simulink model "Amp_baseline"  (R2020a)
settings: Solver=ode45  StartTime=0.0  StopTime=inf  RelTol=1e-3
model workspace (MAT data in the model file):
  cfg_native : object (value not decoded)
  en_add_channels = 1
  host_ip = 2130706433
  host_port = 50223
  local_ip = 2130706433
  local_port = 50224
  num_en_channels = 32
  num_samples = 1
  sample_rate = 250
  serial_number = 'NB-2015.10.93'
undefined symbols (not defined in the file or in its folder): currentCFG_Amp_baseline_UB, UB
libraries: gtecHighspeedLib x7, gUSBamplib x1
settings Model: ModifiedByFormat=g.tec  Creator=g.tec medical engineering  LastModifiedBy=g.tec
settings DataIOCC: LimitDataPoints=on  SaveFormat=Array  ReturnWorkspaceOutputs=off
settings OptimizationCC: BlockReduction=off  BooleanDataType=off  LifeSpan=inf
settings DebuggingCC: SaveWithParameterizedLinksMsg=none  UnderspecifiedInitializationDetection=Classic  MergeDetectMultiDrivingBlocksExec=none  SignalResolutionControl=TryResolveAllWithWarning  FrameProcessingCompatibilityMsg=none  SFUnexpectedBacktrackingDiag=warning  SFNoUnconditionalDefaultTransitionDiag=warning  SFExecutionAtInitializationDiag=none  ArithmeticOperatorsInVariantConditions=warning
settings HardwareCC: ProdBitPerPointer=32  ProdBitPerSizeT=32  ProdBitPerPtrDiffT=32  ProdLargestAtomicFloat=None  ProdIntDivRoundTo=Undefined  ProdEndianess=Unspecified  ProdWordSize=32  ProdHWDeviceType=32-bit Generic  TargetUnknown=on
settings ModelReferenceCC: PropagateSignalLabelsOutOfModel=off
settings SFSimCC: SimUseLocalCustomCode=off  CustomCodeUndefinedFunction=UseInterfaceOnly
settings RTWCC: RTWUseLocalCustomCode=off
settings CodeAppCC: StateflowObjectComments=on
settings GRTTargetCC: TargetLangStandard=C89/C90 (ANSI)
settings ConfigComp: CovMetricSettings=dw  CovHtmlReporting=on  CovSaveCumulativeToWorkspaceVar=on  CovSaveSingleToWorkspaceVar=on  CovExternalEMLEnable=off

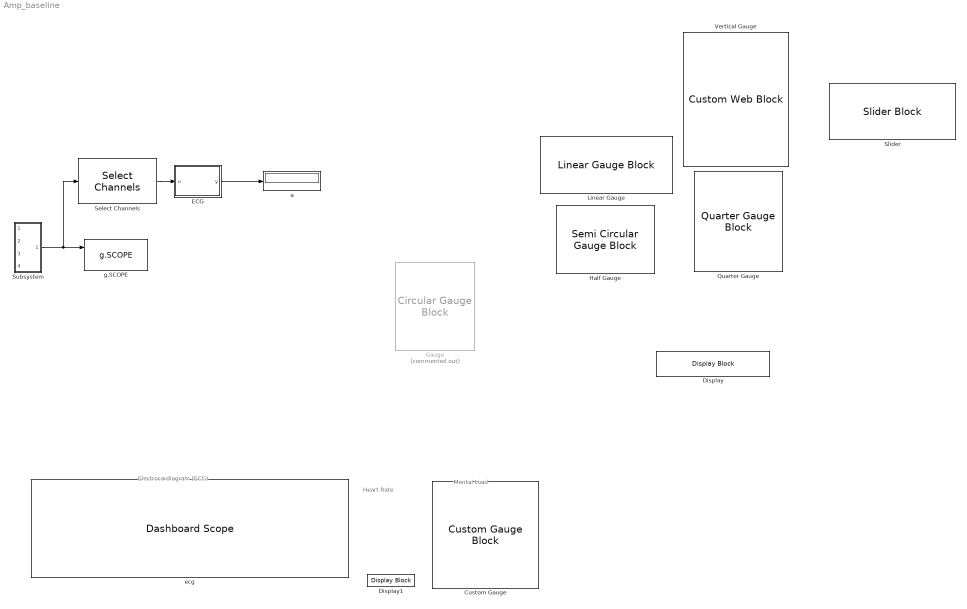
== system Amp_baseline ==
  note: Electrocardiogram (ECG)
  note: .
  note: Heart Rate
  note: Mental Load
  Custom Gauge : CustomGaugeBlock  NeedleImage=data:image/svg+xml;base64,PD94bWwgdmVyc2lvbj0iMS4wIiBlbmNvZGluZz0idXRmLTgiPz4KPCEtLSBHZW5lcmF0b3I6IEFkb2JlIElsbHVzdHJhdG9yIDE5LjIuMSwgU1ZHIEV4cG9ydCBQbHVnLUluIC4gU1ZHIFZlcnNpb246IDYuMDAgQnVpbGQgMCkgIC0tPgo8c3ZnIHZlcnNpb249IjEuMSIgeG1sbnM9Imh0dHA6Ly93d3cudzMub3JnLzIwMDAvc3ZnIiB4bWxuczp4bGluaz0iaHR0cDovL3d3dy53My5vcmcvMTk5OS94bGluayIgeD0iMHB4IiB5PSIwcHgiCgkgdmlld0JveD0iMCAwIDIwMCA1MCIgc3R5bGU9ImVuYWJsZS1iYWNrZ3JvdW5kOm5ldyAw ...(+9940 chars)  NeedleXPos=0.36412625780165153  NeedleYPos=0.47864170306322085  NeedleHeight=0.1316210599644632  NeedleWidth=0.21683597714095698  NeedleInitialRotation=-59.94322499147643  BackgroundImage=data:image/svg+xml;base64,PD94bWwgdmVyc2lvbj0iMS4wIiBlbmNvZGluZz0iVVRGLTgiIHN0YW5kYWxvbmU9Im5vIj8+CjwhLS0gR2VuZXJhdG9yOiBBZG9iZSBJbGx1c3RyYXRvciAxOS4yLjEsIFNWRyBFeHBvcnQgUGx1Zy1JbiAuIFNWRyBWZXJzaW9uOiA2LjAwIEJ1aWxkIDApICAtLT4KCjxzdmcKICAgeG1sbnM6ZGM9Imh0dHA6Ly9wdXJsLm9yZy9kYy9lbGVtZW50cy8xLjEvIgogICB4bWxuczpjYz0iaHR0cDovL2NyZWF0aXZlY29tbW9ucy5vcmcvbnMjIgogICB4bWxuczpyZGY9Imh0dHA6Ly93d3cudzMub3JnLzE5OTkvMDIvMjItcmRmLXN5bnRh ...(+9660 chars)  GaugeMax=1  GaugeArcDefined=true  GaugeArcRadius=0.15412280559666167  GaugeArcStrokeWidth=0.045071457833154936  GaugeArcRotation=240.5385250290321  GaugeArcRatio=0.8333333333333  GaugeArcTransparency=0  ValueArcColor=#1759b0  GaugeTickColor=#faf5c8  ScaleColorsJSON="[{\"Min\":0,\"Max\":0.4,\"Color\":[0.39215686274509803,0.83137254901960778,0.074509803921568626]},{\"Min\":0.4,\"Max\":0.7,\"Color\":[0.92941176470588238,0.69411764705882351,0.12549019607843137]},{\"Min\":0.7,\"Max\":1,\"Color\":[0.996078431372549,0.2,0.0392156862745098]}]"  fixedAspectRatio=on  IsLinearGauge=false  GaugeTrackLeft=0.35  GaugeTrackTop=0.35  GaugeTrackHeight=0.1  GaugeTrackWidth=0.3  GaugeTrackRotation=0
  Display : DisplayBlock  LabelPosition=Hide  Format=short  Transparency=1
  Display1 : DisplayBlock  LabelPosition=Hide  Format=Integer  Transparency=1
  ECG : MATLAB Function  TreatAsAtomicUnit=on
  Gauge : CircularGaugeBlock  Commented=on  ScaleMax=2
  Half Gauge : SemiCircularGaugeBlock
  Linear Gauge : LinearGaugeBlock
  Quarter Gauge : QuarterGaugeBlock
  Select Channels : gtecHighspeedLib/Select Channels  selectedchannels=[2]  totalchannels=14
      settings: SourceProductName=g.HIsys Library
  Slider : SliderBlock
  Subsystem : Subsystem
  Vertical Gauge : CustomWebBlock  ShowInitialText=on  Configuration="{\"components\":[{\"name\":\"LinearScaleComponent\",\"settings\":{\"bounds\":{\"max\":200,\"min\":0,\"tickInterval\":\"auto\"},\"labelColor\":[250,245,199],\"labelFont\":{\"font\":\"Arial\",\"fontSize\":12},\"labelTransparency\":1,\"needleImage\":{\"size\":[21,75],\"src\":\"data:image\\/svg+xml;base64,PHN2ZyB4bWxucz0iaHR0cDovL3d3dy53My5vcmcvMjAwMC9zdmciIHhtbG5zOnhsaW5rPSJodHRwOi8vd3d3LnczLm9yZy8xOTk5L3hsaW5rIiB2aWV3Qm94PSIwIDAgMjEgNzUiPjxkZWZzPjxzdHlsZT4uY2xzLTF7ZmlsbDpub25lO30uY2xzLTJ7aXNvbGF0aW9uOmlzb2xhdGU7fS5jbHMtM3tjbGlwLXBhdGg6dXJsKCNjbGlwLXBhdGgpO30uY2xzLTR7b3BhY2l0eTowLjM7bWl4LWJsZW5kLW1vZGU6bXVsdGlwbHk7fS5jbHMtNXtmaWxsOiNlYjI2Mjk7fTwvc3R5bGU+PGNsaXBQYXRoIGlkPSJjbGlwLXBhdGgiIHRyYW5zZm9y ...(+1928 chars)\",\"srcOrientation\":\"horizontal\"},\"needleOffset\":[-0.01094391244870041,0],\"needleSize\":{\"height\":0.11960078534031414,\"width\":0.7589285714285714},\"position\":[0.002450980392156854,0.07236842105263158,0.7996945488721805,0.9641544117647058],\"scaleColorSize\":0.24,\"scaleColors\":[],\"scaleColorsSize\":0.2,\"tickColor\":[250,245,200],\"tickTransparency\":1,\"valueBarColor\":[23,89,176],\"valueBarSize\":0.23,\"valueBarTransparency\":1}},{\"name\":\"BackgroundImageComponent\",\"settings\":{\"image\":{\"size\":[0,0],\"src\":\"default\",\"srcOrientation\":null},\"position\":[0,0,1,1],\"scaleMode\":\"0\"}}],\"settings\":{\"BindingType\":\"signal\",\"fixedAspectRatio\":\"on\",\"orientation\":\"vertical\"},\"type\":\"LinearGauge\"}"
  a : Display
  ecg : DashboardScope  Tag=ECG  TimeSpan=100  Ymin=0  Ymax=100000  ScaleAtStop=off
  g.SCOPE : gtecHighspeedLib/g.SCOPE
      settings: SourceProductName=g.HIsys Library
  wires:
  Subsystem/1(Out1) -> Select Channels/1, g.SCOPE/1
  Select Channels/1 -> ECG/1(u)
  ECG/1(y) -> a/1

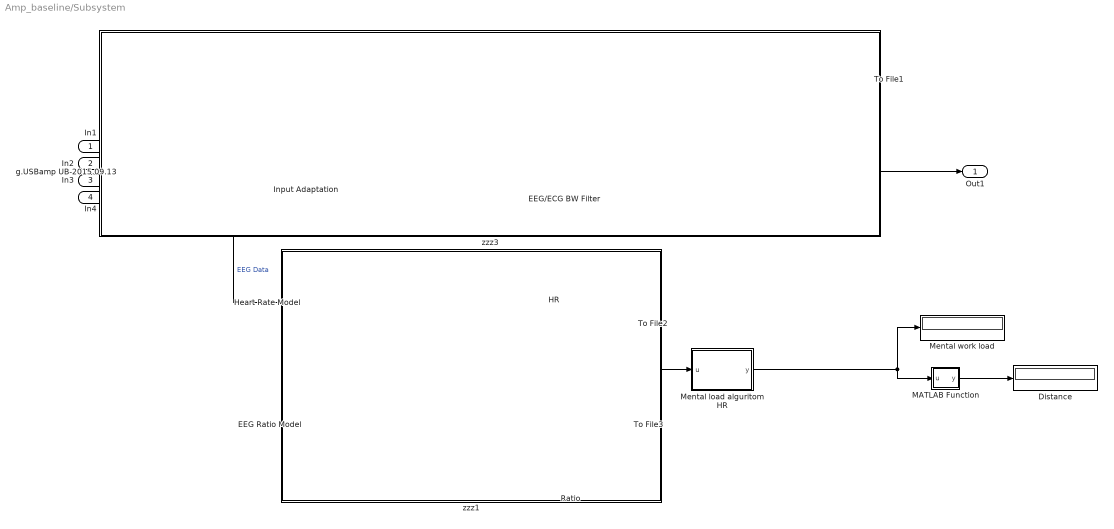
== system Amp_baseline/Subsystem ==
  In1 : Inport
  In2 : Inport  Port=2
  In3 : Inport  Port=3
  In4 : Inport  Port=4
  Distance : Display
  EEG Ratio Model : Subsystem
  EEG/ECG BW Filter : gtecHighspeedLib/EEG//ECG BW Filter  Order=6  LowerFreq=0.1  UpperFreq=30  SampFreq=512
      settings: SourceProductName=g.HIsys Library
  HR : Display
  Heart Rate Model : ModelReference  ModelNameDialog=Heart_Rate_Model_Test  SimulationMode=Normal  ModelReferenceVersion=2.18.00
  Input Adaptation : Subsystem
  MATLAB Function : MATLAB Function  TreatAsAtomicUnit=on
  Mental load alguritom HR : MATLAB Function  TreatAsAtomicUnit=on
  Mental work load : Display
  Ratio : Display
  To File1 : ToFile  Filename=Baseline.mat  MatrixName=Baselinedata
  To File2 : ToFile  Filename=Heartrate_Test.mat  MatrixName=heartRatedata
  To File3 : ToFile  Filename=Ratio.mat  MatrixName=Ratio
  g.USBamp UB-2015.09.13 : gUSBamplib/g.USBamp  cfg=currentCFG_Amp_baseline_UB-2015.09.13.cfg  snr=UB-2015.09.13
      settings: SourceProductName=g.USBamp
  zzz1 : Subsystem  TreatAsAtomicUnit=on
      settings: OpenFcn=% no-op
      mask Display: disp('')
  zzz3 : Subsystem  TreatAsAtomicUnit=on
      settings: OpenFcn=% no-op
      mask Display: disp('')
  Out1 : Outport
  wires:
  g.USBamp UB-2015.09.13/1 -> Input Adaptation/1(In), Heart Rate Model/1, EEG Ratio Model/1(EEG)  "EEG Data"
  EEG/ECG BW Filter/1 -> Out1/1
  Input Adaptation/1(Out) -> To File1/1, EEG/ECG BW Filter/1
  In4/1 -> g.USBamp UB-2015.09.13/4
  In1/1 -> g.USBamp UB-2015.09.13/1
  Heart Rate Model/1 -> Mental load alguritom HR/1(u), HR/1
  EEG Ratio Model/1(Ratio) -> Ratio/1, To File3/1
  Heart Rate Model/2 -> To File2/1
  In3/1 -> g.USBamp UB-2015.09.13/3
  In2/1 -> g.USBamp UB-2015.09.13/2
  MATLAB Function/1(y) -> Distance/1
  Mental load alguritom HR/1(y) -> MATLAB Function/1(u), Mental work load/1

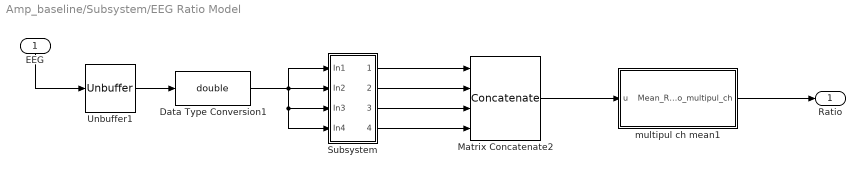
== system Amp_baseline/Subsystem/EEG Ratio Model ==
  EEG : Inport
  Data Type Conversion1 : DataTypeConversion  OutDataTypeStr=double
  Matrix Concatenate2 : Concatenate  NumInputs=4  Mode=Multidimensional array  ConcatenateDimension=2
  Subsystem : Subsystem
  Unbuffer1 : Unbuffer
  multipul ch mean1 : MATLAB Function  TreatAsAtomicUnit=on
  Ratio : Outport
  wires:
  Subsystem/4(Out4) -> Matrix Concatenate2/4
  multipul ch mean1/1(Mean_Ratio_multipul_ch) -> Ratio/1
  Data Type Conversion1/1 -> Subsystem/4(In4), Subsystem/3(In3), Subsystem/1(In1), Subsystem/2(In2)
  Subsystem/3(Out3) -> Matrix Concatenate2/3
  Unbuffer1/1 -> Data Type Conversion1/1
  Matrix Concatenate2/1 -> multipul ch mean1/1(u)
  Subsystem/2(Out2) -> Matrix Concatenate2/2
  Subsystem/1(Out1) -> Matrix Concatenate2/1
  EEG/1 -> Unbuffer1/1

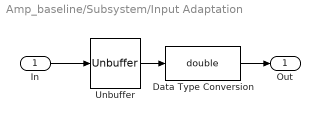
== system Amp_baseline/Subsystem/Input Adaptation ==
  In : Inport
  Data Type Conversion : DataTypeConversion  OutDataTypeStr=double
  Unbuffer : Unbuffer
  Out : Outport
  wires:
  In/1 -> Unbuffer/1
  Unbuffer/1 -> Data Type Conversion/1
  Data Type Conversion/1 -> Out/1

== system Amp_baseline/Subsystem/zzz1 ==

== system Amp_baseline/Subsystem/zzz3 ==

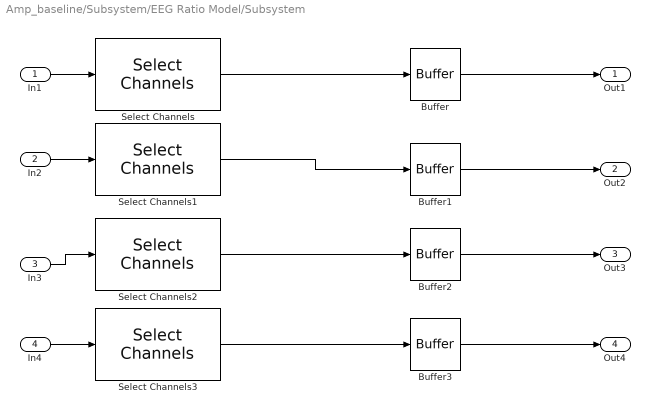
== system Amp_baseline/Subsystem/EEG Ratio Model/Subsystem ==
  In1 : Inport
  In2 : Inport  Port=2
  In3 : Inport  Port=3
  In4 : Inport  Port=4
  Buffer{,1..3} (4 alike) : Buffer  N=2560  OutputFrames=off
  Select Channels : gtecHighspeedLib/Select Channels  selectedchannels=[5]  totalchannels=14
      settings: SourceProductName=g.HIsys Library
  Select Channels1 : gtecHighspeedLib/Select Channels  selectedchannels=[6]  totalchannels=14
      settings: SourceProductName=g.HIsys Library
  Select Channels2 : gtecHighspeedLib/Select Channels  selectedchannels=[7]  totalchannels=14
      settings: SourceProductName=g.HIsys Library
  Select Channels3 : gtecHighspeedLib/Select Channels  selectedchannels=[8]  totalchannels=14
      settings: SourceProductName=g.HIsys Library
  Out1 : Outport
  Out2 : Outport  Port=2
  Out3 : Outport  Port=3
  Out4 : Outport  Port=4
  wires:
  In1/1 -> Select Channels/1
  Select Channels/1 -> Buffer/1
  In2/1 -> Select Channels1/1
  Select Channels1/1 -> Buffer1/1
  Buffer/1 -> Out1/1
  Buffer1/1 -> Out2/1
  Select Channels3/1 -> Buffer3/1
  Buffer3/1 -> Out4/1
  Select Channels2/1 -> Buffer2/1
  In4/1 -> Select Channels3/1
  In3/1 -> Select Channels2/1
  Buffer2/1 -> Out3/1

== matlab function Amp_baseline/Subsystem/Mental load alguritom HR ==
  data: u input; y output
function y = fcn(u)

y= probability_of_mental_howrkload(u);

end

== matlab function Amp_baseline/ECG ==
  data: u input; y output
function y = fcn(u)

y = u;

== matlab function Amp_baseline/Subsystem/EEG Ratio Model/multipul ch mean1 ==
  data: u input; Mean_Ratio_multipul_ch output
function Mean_Ratio_multipul_ch = EEG_Stress_Ratio(u)

   coder.extrinsic('pwelch');
   coder.extrinsic('table2array');
   sampling_rate = 512;
   psd = zeros(513,1);
   frequencies = zeros(513,1);
   
   %initialize an array to store the stress scores for each channel
   stress_scores = zeros(size(u, 2), 1);

   
       for i = 1:size(u, 2)
            
           %extract for current channel
           channel_data = u(:, i);
            
           % Calculate the power spectral density (PSD) of the EEG data
           [psd, frequencies] = pwelch(channel_data, [], [], [], sampling_rate);


           % Calculate the relative power in the alpha frequency band (8-12 Hz)
           alpha_power = sum(psd(frequencies >= 8 & frequencies <= 12)) / sum(psd);

           % Calculate the relative power in the beta frequency band (12-30 Hz)
           beta_power = sum(psd(frequencies >= 12 & frequencies <= 30)) / sum(psd);

           % Calculate the alpha/beta ratio for the current channel
           %alpha_beta_ratio = beta_power / alpha_power ;
           alpha_beta_ratio = log(beta_power) - log(alpha_power) ;
           
           stress_scores(i) = alpha_beta_ratio;      
            
       end
  
    Mean_Ratio_multipul_ch = mean(stress_scores);
end

== matlab function Amp_baseline/Subsystem/MATLAB Function ==
  data: u input; y output
function y = fcn(u)
%#codegen

y = (u*10)+10;
